simulink model "LAB1_Logical"  (R2020b)
settings: Solver=VariableStepAuto  StartTime=0.0  StopTime=10.0  RelTol=1e-3
settings Model: Creator=dssan  LastModifiedBy=dssan

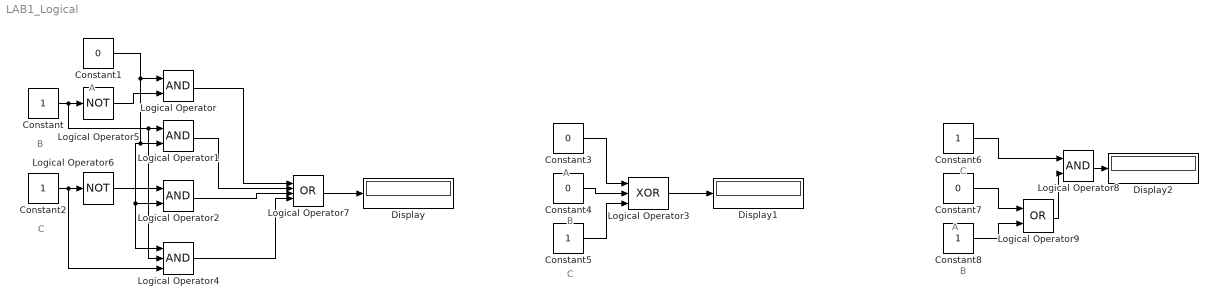
== system LAB1_Logical ==
  note: C
  note: B
  note: A
  note: C
  note: B
  note: A
  note: C
  note: B
  note: A
  Constant{,2,5..6,8} (5 alike) : Constant
  Constant{1,3..4,7} (4 alike) : Constant  Value=0
  Display : Display
  Display1 : Display
  Display2 : Display
  Logical Operator{,1..2,8} (4 alike) : Logic  AllPortsSameDT=off  OutDataTypeStr=boolean
  Logical Operator3 : Logic  Operator=XOR  Inputs=3  AllPortsSameDT=off  OutDataTypeStr=boolean
  Logical Operator4 : Logic  Inputs=3  AllPortsSameDT=off  OutDataTypeStr=boolean
  Logical Operator5 : Logic  Operator=NOT  AllPortsSameDT=off  OutDataTypeStr=boolean
  Logical Operator6 : Logic  Operator=NOT  AllPortsSameDT=off  OutDataTypeStr=boolean
  Logical Operator7 : Logic  Operator=OR  Inputs=4  AllPortsSameDT=off  OutDataTypeStr=boolean
  Logical Operator9 : Logic  Operator=OR  AllPortsSameDT=off  OutDataTypeStr=boolean
  wires:
  Logical Operator6/1 -> Logical Operator2/1
  Logical Operator5/1 -> Logical Operator/2
  Logical Operator/1 -> Logical Operator7/1
  Logical Operator1/1 -> Logical Operator7/2
  Logical Operator2/1 -> Logical Operator7/3
  Logical Operator4/1 -> Logical Operator7/4
  Constant2/1 -> Logical Operator4/3, Logical Operator6/1
  Constant1/1 -> Logical Operator2/2, Logical Operator4/1, Logical Operator1/2, Logical Operator/1
  Constant/1 -> Logical Operator4/2, Logical Operator1/1, Logical Operator5/1
  Logical Operator7/1 -> Display/1
  Constant3/1 -> Logical Operator3/1
  Constant4/1 -> Logical Operator3/2
  Constant5/1 -> Logical Operator3/3
  Logical Operator3/1 -> Display1/1
  Constant8/1 -> Logical Operator9/2
  Constant6/1 -> Logical Operator8/1
  Constant7/1 -> Logical Operator9/1
  Logical Operator9/1 -> Logical Operator8/2
  Logical Operator8/1 -> Display2/1
